simulink model "ChannelEst"  (R2018b)
settings: Solver=FixedStepAuto  StartTime=0  StopTime=500*(15e-9)  FixedStep=15e-9  RelTol=1e-3
settings Model: PauseTimes=160  SnapshotBufferSize=1  SnapshotInterval=1  Creator=jason  LastModifiedBy=jason
settings OptimizationCC: BlockReduction=off  ConditionallyExecuteInputs=off  DefaultParameterBehavior=Inlined
settings DebuggingCC: AlgebraicLoopMsg=error
settings HardwareCC: ProdBitPerPointer=32  ProdBitPerSizeT=32  ProdBitPerPtrDiffT=32  ProdLargestAtomicFloat=None  ProdIntDivRoundTo=Undefined  ProdEndianess=Unspecified  ProdWordSize=32  ProdHWDeviceType=ASIC/FPGA->ASIC/FPGA  TargetBitPerLong=64  TargetBitPerPointer=64  TargetBitPerSizeT=64  TargetBitPerPtrDiffT=64  TargetLongLongMode=on  TargetIntDivRoundTo=Zero  TargetEndianess=LittleEndian  TargetWordSize=64  TargetHWDeviceType=Custom Processor->MATLAB Host Computer  ProdEqTarget=off

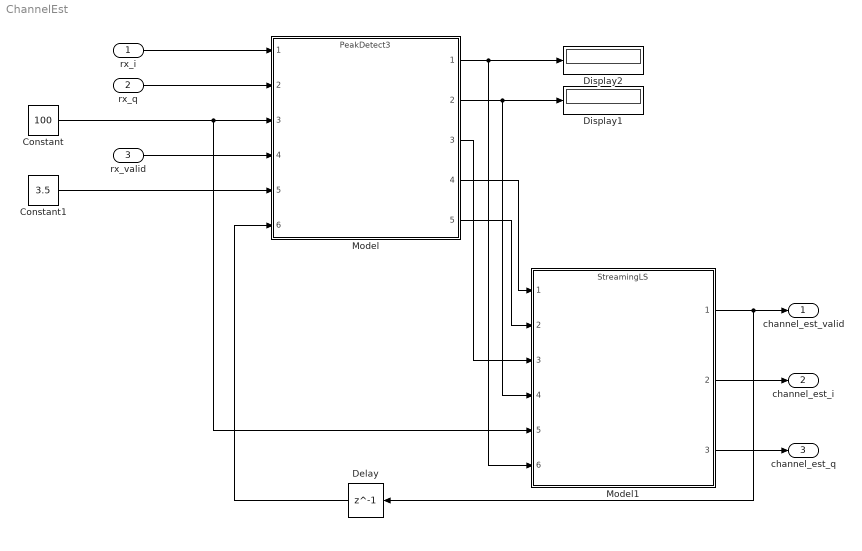
== system ChannelEst ==
  rx_i : Inport  OutDataTypeStr=fixdt(1,16,15)  SampleTime=15e-9
  rx_q : Inport  Port=2  OutDataTypeStr=fixdt(1,16,15)  SampleTime=15e-9
  rx_valid : Inport  Port=3  OutDataTypeStr=boolean  SampleTime=15e-9
  Constant : Constant  Value=100  OutDataTypeStr=uint16  SampleTime=15e-9
  Constant1 : Constant  Value=3.5  OutDataTypeStr=fixdt(1,32,16)  SampleTime=15e-9
  Delay : Delay  DelayLength=1
  Display1 : Display
  Display2 : Display
  Model : ModelReference  ModelNameDialog=PeakDetect3.slx  SimulationMode=Normal  ModelReferenceVersion=1.286
  Model1 : ModelReference  ModelNameDialog=StreamingLS.slx  SimulationMode=Normal  ModelReferenceVersion=1.119
  channel_est_valid : Outport  OutDataTypeStr=boolean
  channel_est_i : Outport  Port=2
  channel_est_q : Outport  Port=3
  wires:
  Model/1 -> Model1/6, Display2/1
  Constant/1 -> Model1/5, Model/3
  rx_valid/1 -> Model/4
  Model/2 -> Model1/4, Display1/1
  rx_q/1 -> Model/2
  rx_i/1 -> Model/1
  Model1/1 -> Delay/1, channel_est_valid/1
  Model1/2 -> channel_est_i/1
  Constant1/1 -> Model/5
  Model1/3 -> channel_est_q/1
  Model/3 -> Model1/3
  Model/4 -> Model1/1
  Model/5 -> Model1/2
  Delay/1 -> Model/6
